simulink model "datatypeconversion_test"  (Simulink 9.0)
settings: Solver=FixedStepAuto  StartTime=0.0  StopTime=10.0  FixedStep=0.1  RelTol=1e-3  EnableMultiTasking=on
settings Model: SuppressorTable=22 serialization::archive 11 0 6 0 0 0 0 0  Creator=arnaud  LastModifiedBy=hbourbou
settings DataIOCC: LimitDataPoints=on  SaveFormat=StructureWithTime  SignalLoggingSaveFormat=ModelDataLogs
settings OptimizationCC: ExpressionDepthLimit=2147483647
settings DebuggingCC: SolverPrmCheckMsg=warning  FcnCallInpInsideContextMsg=warning  StateNameClashWarn=warning
settings GRTTargetCC: GeneratePreprocessorConditionals=Disable all  CombineOutputUpdateFcns=off  GRTInterface=on
settings ConfigComp: CovSFcnEnable=off

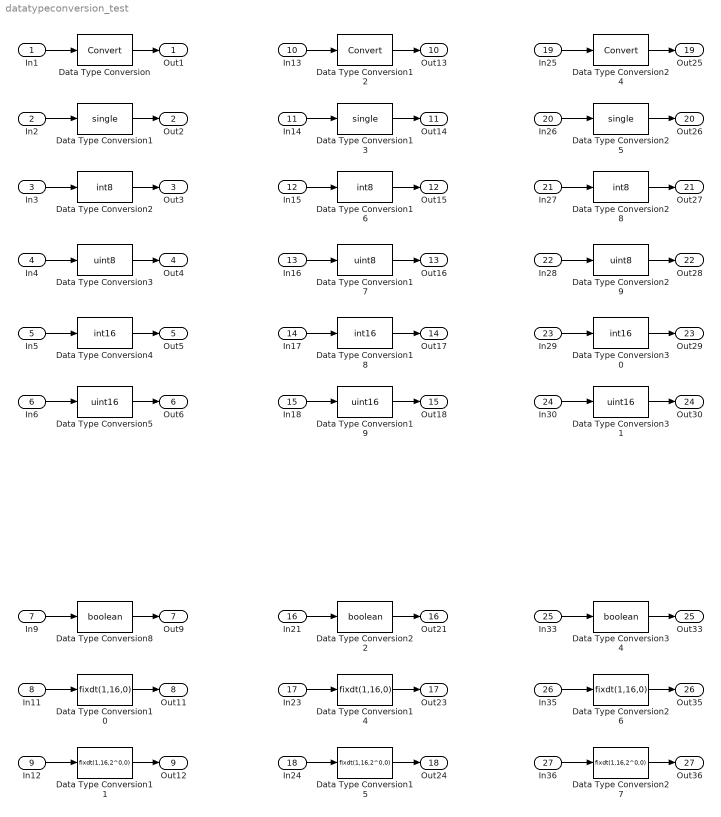
== system datatypeconversion_test ==
  In1 : Inport  OutDataTypeStr=double  PortDimensions=1
  In2 : Inport  Port=2  OutDataTypeStr=double  PortDimensions=1
  In3 : Inport  Port=3  OutDataTypeStr=double  PortDimensions=1
  In4 : Inport  Port=4  OutDataTypeStr=double  PortDimensions=1
  In5 : Inport  Port=5  OutDataTypeStr=double  PortDimensions=1
  In6 : Inport  Port=6  OutDataTypeStr=double  PortDimensions=1
  In9 : Inport  Port=7  OutDataTypeStr=double  PortDimensions=1
  In11 : Inport  Port=8  OutDataTypeStr=double  PortDimensions=1
  In12 : Inport  Port=9  OutDataTypeStr=double  PortDimensions=1
  In13 : Inport  Port=10  OutDataTypeStr=single  PortDimensions=1
  In14 : Inport  Port=11  OutDataTypeStr=single  PortDimensions=1
  In15 : Inport  Port=12  OutDataTypeStr=single  PortDimensions=1
  In16 : Inport  Port=13  OutDataTypeStr=single  PortDimensions=1
  In17 : Inport  Port=14  OutDataTypeStr=single  PortDimensions=1
  In18 : Inport  Port=15  OutDataTypeStr=single  PortDimensions=1
  In21 : Inport  Port=16  OutDataTypeStr=single  PortDimensions=1
  In23 : Inport  Port=17  OutDataTypeStr=single  PortDimensions=1
  In24 : Inport  Port=18  OutDataTypeStr=single  PortDimensions=1
  In25 : Inport  Port=19  OutDataTypeStr=int8  PortDimensions=1
  In26 : Inport  Port=20  OutDataTypeStr=int8  PortDimensions=1
  In27 : Inport  Port=21  OutDataTypeStr=int8  PortDimensions=1
  In28 : Inport  Port=22  OutDataTypeStr=int8  PortDimensions=1
  In29 : Inport  Port=23  OutDataTypeStr=int8  PortDimensions=1
  In30 : Inport  Port=24  OutDataTypeStr=int8  PortDimensions=1
  In33 : Inport  Port=25  OutDataTypeStr=int8  PortDimensions=1
  In35 : Inport  Port=26  OutDataTypeStr=int8  PortDimensions=1
  In36 : Inport  Port=27  OutDataTypeStr=int8  PortDimensions=1
  Data Type Conversion : DataTypeConversion
  Data Type Conversion1 : DataTypeConversion  OutDataTypeStr=single
  Data Type Conversion10 : DataTypeConversion  OutDataTypeStr=fixdt(1,16,0)
  Data Type Conversion11 : DataTypeConversion  OutDataTypeStr=fixdt(1,16,2^0,0)
  Data Type Conversion12 : DataTypeConversion
  Data Type Conversion13 : DataTypeConversion  OutDataTypeStr=single
  Data Type Conversion14 : DataTypeConversion  OutDataTypeStr=fixdt(1,16,0)
  Data Type Conversion15 : DataTypeConversion  OutDataTypeStr=fixdt(1,16,2^0,0)
  Data Type Conversion16 : DataTypeConversion  OutDataTypeStr=int8
  Data Type Conversion17 : DataTypeConversion  OutDataTypeStr=uint8
  Data Type Conversion18 : DataTypeConversion  OutDataTypeStr=int16
  Data Type Conversion19 : DataTypeConversion  OutDataTypeStr=uint16
  Data Type Conversion2 : DataTypeConversion  OutDataTypeStr=int8
  Data Type Conversion22 : DataTypeConversion  OutDataTypeStr=boolean
  Data Type Conversion24 : DataTypeConversion
  Data Type Conversion25 : DataTypeConversion  OutDataTypeStr=single
  Data Type Conversion26 : DataTypeConversion  OutDataTypeStr=fixdt(1,16,0)
  Data Type Conversion27 : DataTypeConversion  OutDataTypeStr=fixdt(1,16,2^0,0)
  Data Type Conversion28 : DataTypeConversion  OutDataTypeStr=int8
  Data Type Conversion29 : DataTypeConversion  OutDataTypeStr=uint8
  Data Type Conversion3 : DataTypeConversion  OutDataTypeStr=uint8
  Data Type Conversion30 : DataTypeConversion  OutDataTypeStr=int16
  Data Type Conversion31 : DataTypeConversion  OutDataTypeStr=uint16
  Data Type Conversion34 : DataTypeConversion  OutDataTypeStr=boolean
  Data Type Conversion4 : DataTypeConversion  OutDataTypeStr=int16
  Data Type Conversion5 : DataTypeConversion  OutDataTypeStr=uint16
  Data Type Conversion8 : DataTypeConversion  OutDataTypeStr=boolean
  Out1 : Outport
  Out2 : Outport  Port=2
  Out3 : Outport  Port=3
  Out4 : Outport  Port=4
  Out5 : Outport  Port=5
  Out6 : Outport  Port=6
  Out9 : Outport  Port=7
  Out11 : Outport  Port=8
  Out12 : Outport  Port=9
  Out13 : Outport  Port=10
  Out14 : Outport  Port=11
  Out15 : Outport  Port=12
  Out16 : Outport  Port=13
  Out17 : Outport  Port=14
  Out18 : Outport  Port=15
  Out21 : Outport  Port=16
  Out23 : Outport  Port=17
  Out24 : Outport  Port=18
  Out25 : Outport  Port=19
  Out26 : Outport  Port=20
  Out27 : Outport  Port=21
  Out28 : Outport  Port=22
  Out29 : Outport  Port=23
  Out30 : Outport  Port=24
  Out33 : Outport  Port=25
  Out35 : Outport  Port=26
  Out36 : Outport  Port=27
  wires:
  Data Type Conversion/1 -> Out1/1
  In1/1 -> Data Type Conversion/1
  Data Type Conversion1/1 -> Out2/1
  In2/1 -> Data Type Conversion1/1
  Data Type Conversion2/1 -> Out3/1
  In3/1 -> Data Type Conversion2/1
  In4/1 -> Data Type Conversion3/1
  Data Type Conversion3/1 -> Out4/1
  Data Type Conversion4/1 -> Out5/1
  In5/1 -> Data Type Conversion4/1
  Data Type Conversion5/1 -> Out6/1
  In6/1 -> Data Type Conversion5/1
  In9/1 -> Data Type Conversion8/1
  Data Type Conversion8/1 -> Out9/1
  In11/1 -> Data Type Conversion10/1
  Data Type Conversion10/1 -> Out11/1
  In12/1 -> Data Type Conversion11/1
  Data Type Conversion11/1 -> Out12/1
  Data Type Conversion12/1 -> Out13/1
  In13/1 -> Data Type Conversion12/1
  Data Type Conversion13/1 -> Out14/1
  In14/1 -> Data Type Conversion13/1
  Data Type Conversion16/1 -> Out15/1
  In15/1 -> Data Type Conversion16/1
  In16/1 -> Data Type Conversion17/1
  Data Type Conversion17/1 -> Out16/1
  Data Type Conversion18/1 -> Out17/1
  In17/1 -> Data Type Conversion18/1
  Data Type Conversion19/1 -> Out18/1
  In18/1 -> Data Type Conversion19/1
  In21/1 -> Data Type Conversion22/1
  Data Type Conversion22/1 -> Out21/1
  In23/1 -> Data Type Conversion14/1
  Data Type Conversion14/1 -> Out23/1
  In24/1 -> Data Type Conversion15/1
  Data Type Conversion15/1 -> Out24/1
  Data Type Conversion24/1 -> Out25/1
  In25/1 -> Data Type Conversion24/1
  Data Type Conversion25/1 -> Out26/1
  In26/1 -> Data Type Conversion25/1
  Data Type Conversion28/1 -> Out27/1
  In27/1 -> Data Type Conversion28/1
  In28/1 -> Data Type Conversion29/1
  Data Type Conversion29/1 -> Out28/1
  Data Type Conversion30/1 -> Out29/1
  In29/1 -> Data Type Conversion30/1
  Data Type Conversion31/1 -> Out30/1
  In30/1 -> Data Type Conversion31/1
  In33/1 -> Data Type Conversion34/1
  Data Type Conversion34/1 -> Out33/1
  In35/1 -> Data Type Conversion26/1
  Data Type Conversion26/1 -> Out35/1
  In36/1 -> Data Type Conversion27/1
  Data Type Conversion27/1 -> Out36/1
